simulink model "frdc_ut"  (Simulink 8.1)
settings: Solver=FixedStepDiscrete  StartTime=0.0  StopTime=Inf  FixedStep=0.005  RelTol=1e-3
PostLoadFcn:
  | , if any(exist('dsrtsu_mdlpostloadfcn', 'file') == [2, 3, 6]), try dsrtsu_mdlpostloadfcn('Execute', bdroot); catch fprintf('Error in PostLoadFcn (dsrtsu_mdlpostloadfcn) for model "%s":\n %s\n', bdroot, lasterr); end, end,
libraries: frdc x1
settings Model: DSRTSU_INTERNAL_RTI_VER=450  DSRTSU_INTERNAL_RTI_TYPE=rti1401  RTICANMMDATA=struct('GeneralSetupData',struct('modelroot','D:\ELN150201_TAIWAN\trunk\AdasDragon\software\sw_development\arch\app\jud','generalsettings',struct('filesettings',struct('destfolder',struct('Name','RTICANMM_FILES','Check',1),'buildfolder',struct('Name','.','Check',1),'AbsDestfolder',struct('Name','D:\ELN150201_TAIWAN\trunk\AdasDragon\software\sw_development\arch\app\jud\RTICANMM_FILES'),'AbsBuildfolder',struct('Name','D:\ELN150201_TAIWAN\trunk\AdasDragon\software\sw_development\arch\app\jud'))),'options',struct('addpaths',1,'rmpaths',1,'addtrcexclusion',logical(1),'cannavigator',struct('checkmonitoring',0),'show_usrtrc',0,'use_usrtrc',0),'advanced',struct('options',[1 1 1 1 1 1 1 1 1 1 1 1 1 1 1 1 1 1 1 1 1 1 1 1 1 1 1 1 1 1 1 1 1 1 1 1 1 1 1 1 1 1 1 1 1 1 1 1 1 1 1 1 1 1 1 1 1 1 1 1 1 1 1 1 1 1 1 1 1 1 1 1 1 1 1 1 1 1 1 1 1 1 1 1 1 1 1 1 1 1 1 1 1 1 1 1 1 1 1 1]),'MPSetup',{{}},'modelname','frdc_ut','block','frdc_ut'))  DSRTSU_INTERNAL_RTIFPGA=40  Creator=tescamilla  LastModifiedBy=AT015555  BufferReuse=off
settings DataIOCC: SignalLoggingSaveFormat=Dataset
settings OptimizationCC: BlockReduction=off  OptimizeBlockIOStorage=off  BufferReuse=off  ExpressionFolding=off  ExpressionDepthLimit=128  LocalBlockOutputs=off
settings DebuggingCC: FcnCallInpInsideContextMsg=EnableAllAsError
settings HardwareCC: ProdIntDivRoundTo=Zero  ProdEndianess=BigEndian  ProdHWDeviceType=Generic->Custom  TargetIntDivRoundTo=Zero  TargetEndianess=BigEndian  TargetHWDeviceType=Generic->Custom
settings RTWCC: SystemTargetFile=rti1401.tlc  MakeCommand=make_rti  TemplateMakefile=rti1401.tmf  Description=dSPACE DS1401 Hardware Platform  ProcessScript=rti1401_make_rtw_hook
settings STFCustomTargetCC: CodeReplacementLibrary=ANSI_C  ParMdlRefBuildCompliant=on  GeneratePreprocessorConditionals=Disable all  MatFileLogging=on  SystemTargetFile=rti1401.tlc
settings GRTTargetCC: CompOptLevelCompliant=off  ConcurrentExecutionCompliant=off  ExtModeMexFile=noextcomm
settings CustomProperty: DataType=RTWOptions_EnumType_C__Program Files (x86)_dSPACE RCPHIL 2014-B_MATLAB_RTI_RTI1401_TLC_rti1401_1InitialSimState  Value=RUN
settings EnumStrPairs: String=RUN

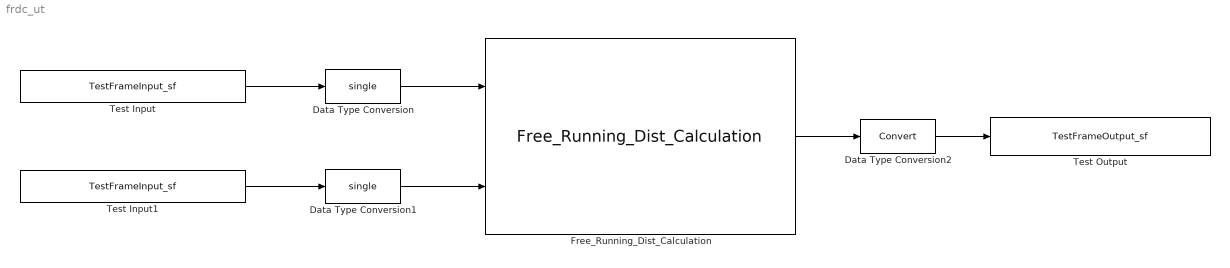
== system frdc_ut ==
  Data Type Conversion : DataTypeConversion  OutDataTypeStr=single
  Data Type Conversion1 : DataTypeConversion  OutDataTypeStr=single
  Data Type Conversion2 : DataTypeConversion
  Free_Running_Dist_Calculation : frdc/Free_Running_Dist_Calculation
  Test Input : S-Function  FunctionName=TestFrameInput_sf  Parameters=varname,sampletime  EnableBusSupport=off  mask(Test Input){varname=FreeRunningTime_sec, sampletime=0.005}
      mask prompts: varname "Name:"; sampletime "Sample Time:"
      mask help: Outputs the value of a Test Input variable from an Excel spreadsheet when used with the runsiltest script. Otherwise outputs 0.
      mask Display: fprintf('Test Input:\n%s',varname);
  Test Input1 : S-Function  FunctionName=TestFrameInput_sf  Parameters=varname,sampletime  EnableBusSupport=off  mask(Test Input){varname=VehSpd_mps, sampletime=0.005}
      mask prompts: varname "Name:"; sampletime "Sample Time:"
      mask help: Outputs the value of a Test Input variable from an Excel spreadsheet when used with the runsiltest script. Otherwise outputs 0.
      mask Display: fprintf('Test Input:\n%s',varname);
  Test Output : S-Function  FunctionName=TestFrameOutput_sf  Parameters=varname,sampletime  EnableBusSupport=off  mask(Test Output){varname=FreeRunningDist_m, sampletime=-1}
      mask prompts: varname "Name:"; sampletime "Sample Time:"
      mask help: Samples the value of a Test Output variable from an Excel spreadsheet when used with the runsiltest script. Otherwise does nothing.
      mask Display: fprintf('Test Output:\n%s',varname);
  wires:
  Free_Running_Dist_Calculation/1 -> Data Type Conversion2/1
  Data Type Conversion2/1 -> Test Output/1
  Test Input/1 -> Data Type Conversion/1
  Data Type Conversion/1 -> Free_Running_Dist_Calculation/1
  Test Input1/1 -> Data Type Conversion1/1
  Data Type Conversion1/1 -> Free_Running_Dist_Calculation/2
